simulink model "three_models_observer"  (R2021b)
settings: Solver=ode45  StartTime=0.0  StopTime=50  FixedStep=0.01  RelTol=1e-6  EnableMultiTasking=on
values from neighbouring files (symbols this model uses):
  a = -l^2+J/(mc+mp)    (= 0.00589092533208)    [parameters.m]    (also in simulation_models.m)
  A = [0 0 1 0;0 0 0 1;0 -l*mu*g/J -a*Fc/J -l*fp/J;0 -mu*g/J -l*Fc/J -fp/J]    [simulation_models.m]
  A1 = expm(A(2:4,2:4)*0.01)    [simulation_models.m]
  B = [0;0;a/J;l/J]    [simulation_models.m]
  B1 = (A1-eye(3))*inv(A(2:4,2:4))*B(2:4)    [simulation_models.m]
  C = [1 0 0 0;0 1 0 0;0 0 1 0;0 0 0 1]    [simulation_models.m]
  D = [0;0;0;0]    [simulation_models.m]
  DZcp = 6.8    [parameters.m]    (also in simulation_models.m)
  DZcv = 0.08    [parameters.m]    (also in simulation_models.m)
  DZu = 0.4    [parameters.m]    (also in simulation_models.m)
  Fc = 0.75    [parameters.m]    (also in simulation_models.m)
  FCD = 0.2501    [parameters.m]    (also in simulation_models.m)
  FCU = 0.8793    [parameters.m]    (also in simulation_models.m)
  fp = 0.0038    [parameters.m]    (also in simulation_models.m)
  FS = 2    [parameters.m]    (also in simulation_models.m)
  FSD = 2.7457    [parameters.m]    (also in simulation_models.m)
  FSdl = -1    [parameters.m]    (also in simulation_models.m)
  FSU = 2.7972    [parameters.m]    (also in simulation_models.m)
  FSul = 2    [parameters.m]    (also in simulation_models.m)
  g = 9.81    [parameters.m]    (also in simulation_models.m)
  J = 0.0075    [parameters.m]    (also in simulation_models.m)
  l = 0.0167903    [parameters.m]    (also in simulation_models.m)
  M = 22.304    [parameters.m]    (also in simulation_models.m)
  mu = l*(mc+mp)    (= 0.0204002145)    [parameters.m]    (also in simulation_models.m)
  Um = 0.5    [parameters.m]    (also in simulation_models.m)
  Xc = 2    [parameters.m]    (also in simulation_models.m)
  Yc = 2    [parameters.m]    (also in simulation_models.m)
undefined symbols (not defined in the file or in its folder): den, DiscIntNeverNeededParam, num
settings Model: Creator=ramon_perez  LastModifiedBy=szmis
settings SolverCC: AlgebraicLoopSolver=TrustRegion
settings DataIOCC: SaveFormat=Array  SignalLoggingSaveFormat=ModelDataLogs  ReturnWorkspaceOutputs=off
settings OptimizationCC: BlockReduction=off  BooleanDataType=off  ExpressionDepthLimit=2147483647  LifeSpan=inf
settings DebuggingCC: SaveWithParameterizedLinksMsg=none  UnderspecifiedInitializationDetection=Classic  MergeDetectMultiDrivingBlocksExec=none  SignalResolutionControl=TryResolveAllWithWarning  MultiTaskDSMMsg=warning  MultiTaskCondExecSysMsg=none  FcnCallInpInsideContextMsg=warning  StateNameClashWarn=warning  SFUnexpectedBacktrackingDiag=warning  SFNoUnconditionalDefaultTransitionDiag=warning  SFExecutionAtInitializationDiag=none  SFMachineParentedDataDiag=warning  ArithmeticOperatorsInVariantConditions=warning
settings HardwareCC: ProdBitPerPointer=32  ProdBitPerSizeT=32  ProdBitPerPtrDiffT=32  ProdLargestAtomicFloat=None  ProdIntDivRoundTo=Undefined  ProdEndianess=Unspecified  ProdWordSize=32  ProdHWDeviceType=32-bit Generic  TargetUnknown=on
settings ModelReferenceCC: PropagateSignalLabelsOutOfModel=off
settings SFSimCC: SimUseLocalCustomCode=off  CustomCodeUndefinedFunction=UseInterfaceOnly
settings RTWCC: RTWUseLocalCustomCode=off
settings CodeAppCC: StateflowObjectComments=on
settings GRTTargetCC: TargetLangStandard=C89/C90 (ANSI)  CombineOutputUpdateFcns=off  GRTInterface=on
settings ConfigComp: CovMetricSettings=dw  CovSaveCumulativeToWorkspaceVar=on  CovSaveSingleToWorkspaceVar=on  CovExternalEMLEnable=off

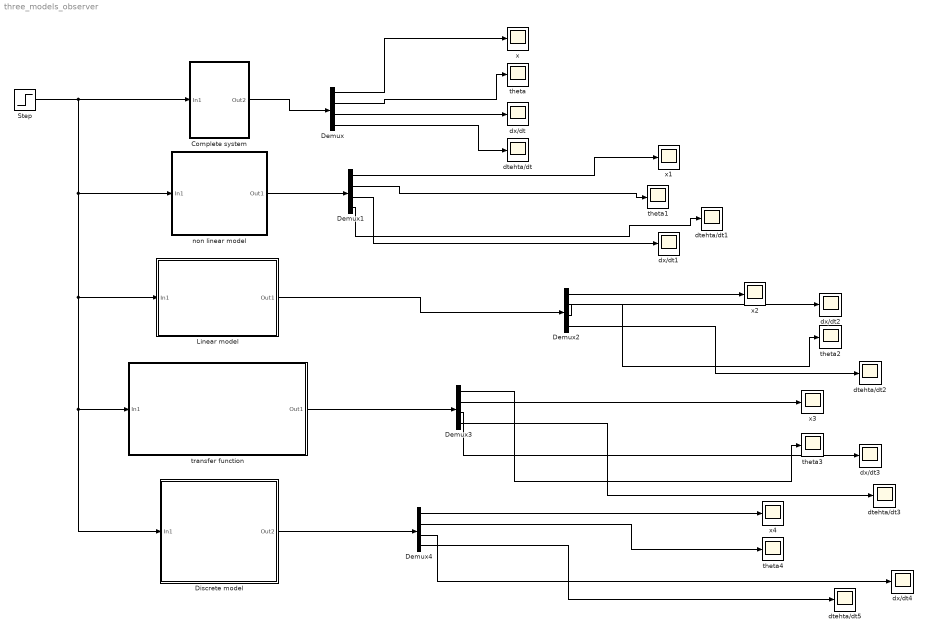
== system three_models_observer ==
  Complete system : Subsystem
  Demux{,1..4} (5 alike) : Demux
  Discrete model : Subsystem
  Linear model : Subsystem
  Step : Step  After=0.3  SampleTime=0
  dtehta/dt{,1..3,5} (5 alike) : Scope
  dx/dt{,1..4} (5 alike) : Scope
  non linear model : Subsystem
  theta{,1..4} (5 alike) : Scope
  transfer function : Subsystem
  x{,1..4} (5 alike) : Scope
  wires:
  Step/1 -> Complete system/1(In1), transfer function/1(In1), Discrete model/1(In1), Linear model/1(In1), non linear model/1(In1)
  Complete system/1(Out2) -> Demux/1
  Demux/1 -> x/1
  Demux/2 -> theta/1
  Demux/3 -> dx/dt/1
  Demux/4 -> dtehta/dt/1
  non linear model/1(Out1) -> Demux1/1
  Demux1/1 -> x1/1
  Demux1/2 -> theta1/1
  Demux1/3 -> dx/dt1/1
  Demux1/4 -> dtehta/dt1/1
  Linear model/1(Out1) -> Demux2/1
  Demux2/1 -> x2/1
  Demux2/2 -> theta2/1
  Demux2/3 -> dx/dt2/1
  Demux2/4 -> dtehta/dt2/1
  Demux3/1 -> x3/1
  Demux3/2 -> theta3/1
  Demux3/3 -> dx/dt3/1
  Demux3/4 -> dtehta/dt3/1
  transfer function/1(Out1) -> Demux3/1
  Demux4/1 -> x4/1
  Demux4/2 -> theta4/1
  Demux4/3 -> dx/dt4/1
  Demux4/4 -> dtehta/dt5/1
  Discrete model/1(Out2) -> Demux4/1

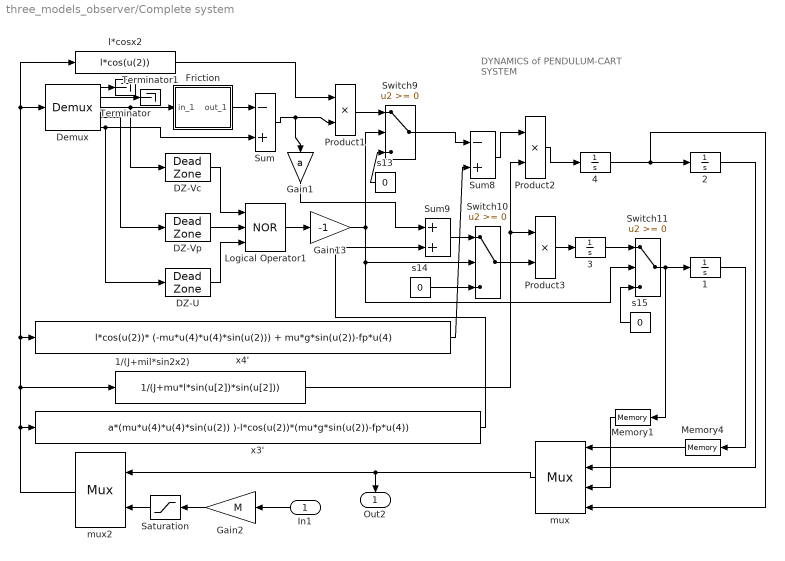
== system three_models_observer/Complete system ==
  note: DYNAMICS
      | of
      | PENDULUM-CART SYSTEM
  In1 : Inport
  1 : Integrator
  1/(J+mil*sin2x2) : Fcn  Expr=1/(J+mu*l*sin(u[2])*sin(u[2]))
  2 : Integrator  InitialCondition=pi
  3 : Integrator
  4 : Integrator
  DZ-U : DeadZone  LowerValue=-DZu  UpperValue=DZu  SaturateOnIntegerOverflow=on
  DZ-Vc : DeadZone  LowerValue=-DZcv  UpperValue=DZcv  SaturateOnIntegerOverflow=on
  DZ-Vp : DeadZone  LowerValue=-DZcp  UpperValue=DZcp  SaturateOnIntegerOverflow=on
  Demux : Demux  Outputs=5
      settings: DisplayOption=none
  Friction : Subsystem  mask(Friction model){FSD=FSD, FSU=FSU, FCD=FCD, FCU=FCU, FSdl=FSdl, FSul=FSul, FS=FS, Xc=Xc, Yc=Yc, small=DZcv}
      mask prompts: FSD "Static friction (FSD) [N]:"; FSU "Static friction (FSU) [N] :"; FCD "Columbic friction (FCD) [N]:"; FCU "Coulombic friction (FCU)  [N] :"; FSdl "Coulombic friction (FSdl) [N]:"; FSul "Coulombic friction (Fsul) [N]:"; FS "Coulombic friction (FS) [N]:"; Xc "Point for minimum (X1) [m/s] :"; Yc "Friction value for Xc point (Yc) [N] :"; small "Linear zone :"
      mask help: Friction implemented as nonlinear function. Copyright Adam PI£AT 1997.
      mask init:
      | Z=small;
      mask Help: Friction vs. cart velocity
      mask Display: plot(0,0,10,20,[1,9],[10,10],[5,5],[1,19],[0,1,2,3,4,5],[7,7.5,8,8.5,8.3,3],[5,6,7,8,9,10],[17,11.7,11.5,12,12.5,13])
  Gain1 : Gain  Gain=a  SaturateOnIntegerOverflow=on  OutDataTypeStr=Inherit: Same as input  ParamDataTypeStr=Inherit: Same as input
  Gain13 : Gain  Gain=-1  SaturateOnIntegerOverflow=on  OutDataTypeStr=Inherit: Same as input  ParamDataTypeStr=Inherit: Same as input
  Gain2 : Gain  Gain=M  OutDataTypeStr=Inherit: Same as input  ParamDataTypeStr=Inherit: Same as input
  Logical Operator1 : Logic  Operator=NOR  Inputs=3
  Memory1 : Memory
  Memory4 : Memory
  Product1 : Product  InputSameDT=on  RndMeth=Zero  SaturateOnIntegerOverflow=on  OutDataTypeStr=Inherit: Same as first input
  Product2 : Product  InputSameDT=on  RndMeth=Zero  SaturateOnIntegerOverflow=on  OutDataTypeStr=Inherit: Same as first input
  Product3 : Product  InputSameDT=on  RndMeth=Zero  SaturateOnIntegerOverflow=on  OutDataTypeStr=Inherit: Same as first input
  Saturation : Saturate  UpperLimit=Um*M  LowerLimit=-Um*M
  Sum : Sum  Inputs=-+  InputSameDT=on  SaturateOnIntegerOverflow=on  OutDataTypeStr=Inherit: Same as first input
  Sum8 : Sum  Inputs=-+  InputSameDT=on  SaturateOnIntegerOverflow=on  OutDataTypeStr=Inherit: Same as first input
  Sum9 : Sum  InputSameDT=on  SaturateOnIntegerOverflow=on  OutDataTypeStr=Inherit: Same as first input
  Switch10 : Switch  SaturateOnIntegerOverflow=on  InputSameDT=on
  Switch11 : Switch  SaturateOnIntegerOverflow=on  InputSameDT=on
  Switch9 : Switch  SaturateOnIntegerOverflow=on  InputSameDT=on
  Terminator : Terminator
  Terminator1 : Terminator
  l*cosx2 : Fcn  Expr=l*cos(u(2))
  mux : Mux
  mux2 : Mux  Inputs=[4 1]
  s13 : Constant  Value=0
  s14 : Constant  Value=0
  s15 : Constant  Value=0
  x3' : Fcn  Expr=a*(mu*u(4)*u(4)*sin(u(2)) )-l*cos(u(2))*(mu*g*sin(u(2))-fp*u(4))
  x4' : Fcn  Expr=l*cos(u(2))* (-mu*u(4)*u(4)*sin(u(2))) + mu*g*sin(u(2))-fp*u(4)
  Out2 : Outport
  wires:
  Demux/2 -> Terminator1/1
  Demux/1 -> Terminator/1
  l*cosx2/1 -> Product1/1
  DZ-U/1 -> Logical Operator1/3
  DZ-Vp/1 -> Logical Operator1/2
  DZ-Vc/1 -> Logical Operator1/1
  Logical Operator1/1 -> Gain13/1
  s13/1 -> Switch9/3
  Switch9/1 -> Sum8/1
  s14/1 -> Switch10/3
  Product1/1 -> Switch9/1
  x4'/1 -> Sum8/2
  Sum8/1 -> Product2/1
  Product2/1 -> 4/1
  Product3/1 -> 3/1
  Demux/3 -> Friction/1(in_1), DZ-Vc/1
  Demux/4 -> DZ-Vp/1
  Sum9/1 -> Switch10/1
  s15/1 -> Switch11/3
  Memory1/1 -> mux/3
  Switch11/1 -> 1/1, Memory1/1
  Saturation/1 -> mux2/2
  Gain2/1 -> Saturation/1
  Friction/1(out_1) -> Sum/1
  Gain13/1 -> Switch9/2, Switch11/2, Switch10/2
  Demux/5 -> Sum/2, DZ-U/1
  Switch10/1 -> Product3/2
  Sum/1 -> Product1/2, Gain1/1
  Gain1/1 -> Sum9/1
  mux2/1 -> x3'/1, l*cosx2/1, Demux/1, x4'/1, 1/(J+mil*sin2x2)/1
  x3'/1 -> Sum9/2
  1/(J+mil*sin2x2)/1 -> Product2/2, Product3/1
  1/1 -> Memory4/1
  Memory4/1 -> mux/1
  4/1 -> 2/1, mux/4
  3/1 -> Switch11/1
  In1/1 -> Gain2/1
  mux/1 -> mux2/1, Out2/1
  2/1 -> mux/2

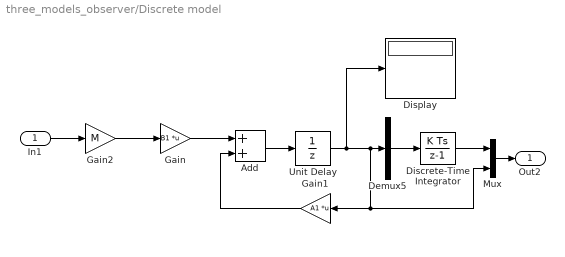
== system three_models_observer/Discrete model ==
  In1 : Inport
  Add : Sum
  Demux5 : Demux  Outputs=3
  Discrete-Time Integrator : DiscreteIntegrator  SampleTime=0.1  ICPrevOutput=DiscIntNeverNeededParam  ICPrevScaledInput=DiscIntNeverNeededParam
  Display : Display
  Gain : Gain  Gain=B1  Multiplication=Matrix(K*u)  SampleTime=0.1
  Gain1 : Gain  Gain=A1  Multiplication=Matrix(K*u)  SampleTime=0.1
  Gain2 : Gain  Gain=M  SampleTime=0.1
  Mux : Mux  Inputs=2
  Unit Delay : UnitDelay  SampleTime=0.1  HasFrameUpgradeWarning=on
  Out2 : Outport
  wires:
  Add/1 -> Unit Delay/1
  Gain/1 -> Add/1
  Gain1/1 -> Add/2
  Unit Delay/1 -> Display/1, Demux5/1, Gain1/1, Mux/2
  Gain2/1 -> Gain/1
  Discrete-Time Integrator/1 -> Mux/1
  Demux5/2 -> Discrete-Time Integrator/1
  In1/1 -> Gain2/1
  Mux/1 -> Out2/1

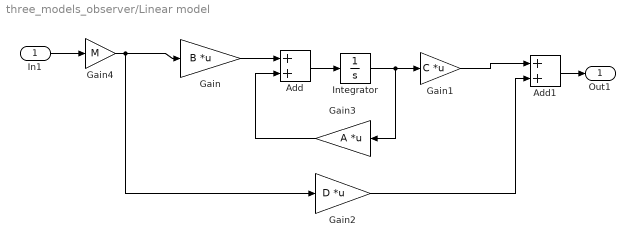
== system three_models_observer/Linear model ==
  In1 : Inport
  Add : Sum
  Add1 : Sum
  Gain : Gain  Gain=B  Multiplication=Matrix(K*u)
  Gain1 : Gain  Gain=C  Multiplication=Matrix(K*u)
  Gain2 : Gain  Gain=D  Multiplication=Matrix(K*u)
  Gain3 : Gain  Gain=A  Multiplication=Matrix(K*u)
  Gain4 : Gain  Gain=M
  Integrator : Integrator
  Out1 : Outport
  wires:
  Add/1 -> Integrator/1
  Gain/1 -> Add/1
  Gain3/1 -> Add/2
  Integrator/1 -> Gain1/1, Gain3/1
  Gain1/1 -> Add1/1
  Gain2/1 -> Add1/2
  Gain4/1 -> Gain/1, Gain2/1
  In1/1 -> Gain4/1
  Add1/1 -> Out1/1

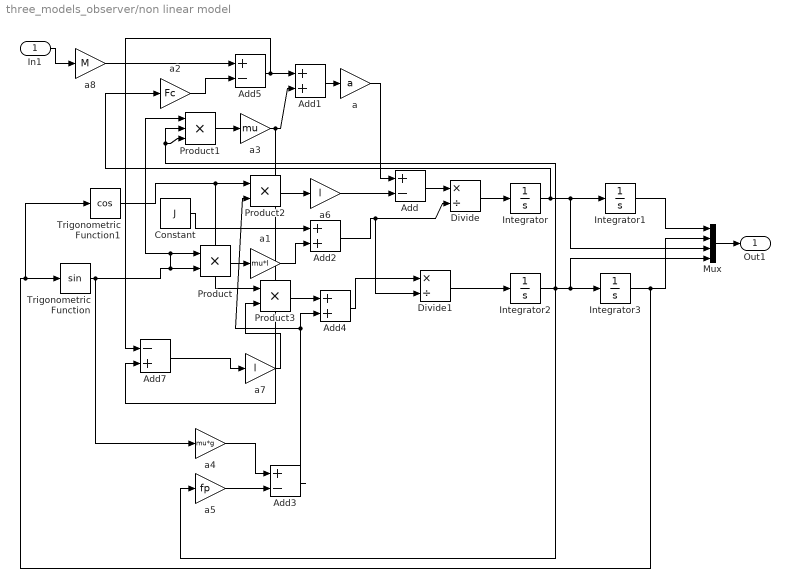
== system three_models_observer/non linear model ==
  In1 : Inport
  Add : Sum  Inputs=+-
  Add1 : Sum
  Add2 : Sum
  Add3 : Sum  Inputs=+-
  Add4 : Sum
  Add5 : Sum  Inputs=+-
  Add7 : Sum  Inputs=-+
  Constant : Constant  Value=J
  Divide : Product  Inputs=*/
  Divide1 : Product  Inputs=*/
  Integrator : Integrator
  Integrator1 : Integrator
  Integrator2 : Integrator
  Integrator3 : Integrator  InitialCondition=pi
  Mux : Mux
  Product : Product  RndMeth=Zero
  Product1 : Product  Inputs=3  RndMeth=Zero
  Product2 : Product  RndMeth=Zero
  Product3 : Product  RndMeth=Zero
  Trigonometric Function : Trigonometry
  Trigonometric Function1 : Trigonometry  Operator=cos
  a : Gain  Gain=a
  a1 : Gain  Gain=mu*l
  a2 : Gain  Gain=Fc
  a3 : Gain  Gain=mu
  a4 : Gain  Gain=mu*g
  a5 : Gain  Gain=fp
  a6 : Gain  Gain=l
  a7 : Gain  Gain=l
  a8 : Gain  Gain=M
  Out1 : Outport
  wires:
  Integrator/1 -> Integrator1/1, Mux/3, a2/1
  Integrator2/1 -> Integrator3/1, Mux/4, Product1/2, Product1/3, a5/1
  Integrator1/1 -> Mux/1
  Integrator3/1 -> Mux/2, Trigonometric Function/1, Trigonometric Function1/1
  Divide1/1 -> Integrator2/1
  Divide/1 -> Integrator/1
  a/1 -> Add/1
  Add/1 -> Divide/1
  Add1/1 -> a/1
  Add2/1 -> Divide/2, Divide1/2
  Constant/1 -> Add2/1
  Trigonometric Function/1 -> Product/2, Product/1, Product1/1, a4/1
  a1/1 -> Add2/2
  Product1/1 -> a3/1
  a3/1 -> Add1/2, Add7/2
  Add4/1 -> Divide1/1
  Add3/1 -> Add4/2, Product2/2
  a4/1 -> Add3/1
  a5/1 -> Add3/2
  Product/1 -> a1/1
  Add5/1 -> Add1/1, Add7/1
  a2/1 -> Add5/2
  a6/1 -> Add/2
  Product2/1 -> a6/1
  Trigonometric Function1/1 -> Product2/1, Product3/1
  Add7/1 -> a7/1
  Product3/1 -> Add4/1
  a7/1 -> Product3/2
  In1/1 -> a8/1
  Mux/1 -> Out1/1
  a8/1 -> Add5/1

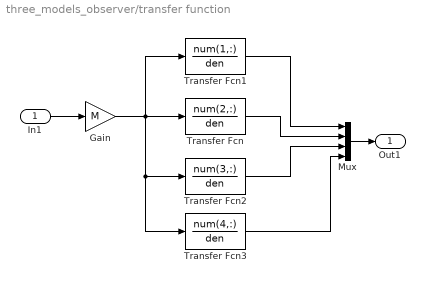
== system three_models_observer/transfer function ==
  In1 : Inport
  Gain : Gain  Gain=M
  Mux : Mux
  Transfer Fcn : TransferFcn  Numerator=num(2,:)  Denominator=den
  Transfer Fcn1 : TransferFcn  Numerator=num(1,:)  Denominator=den
  Transfer Fcn2 : TransferFcn  Numerator=num(3,:)  Denominator=den
  Transfer Fcn3 : TransferFcn  Numerator=num(4,:)  Denominator=den
  Out1 : Outport
  wires:
  Gain/1 -> Transfer Fcn3/1, Transfer Fcn2/1, Transfer Fcn1/1, Transfer Fcn/1
  Transfer Fcn1/1 -> Mux/1
  Transfer Fcn/1 -> Mux/2
  Transfer Fcn2/1 -> Mux/3
  Transfer Fcn3/1 -> Mux/4
  In1/1 -> Gain/1
  Mux/1 -> Out1/1

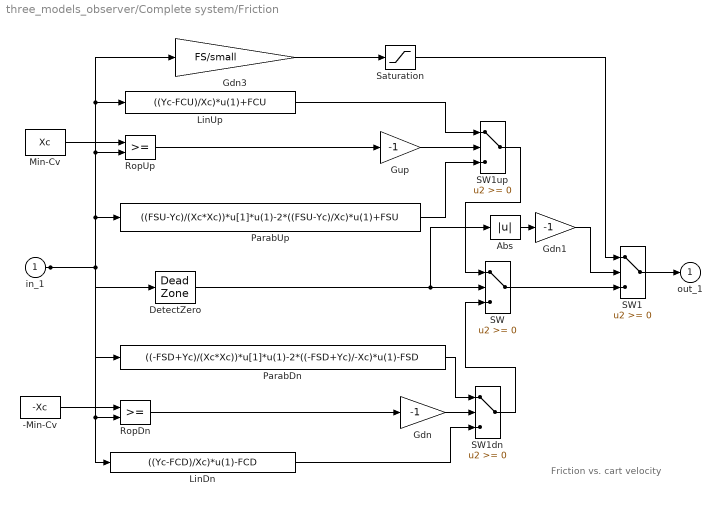
== system three_models_observer/Complete system/Friction ==
  note: Friction vs. cart velocity
  in_1 : Inport
  -Min-Cv : Constant  Value=-Xc
  Abs : Abs  SaturateOnIntegerOverflow=on
  DetectZero : DeadZone  LowerValue=-Z  UpperValue=Z  SaturateOnIntegerOverflow=on
  Gdn : Gain  Gain=-1  SaturateOnIntegerOverflow=on  OutDataTypeStr=Inherit: Same as input  ParamDataTypeStr=Inherit: Same as input
  Gdn1 : Gain  Gain=-1  SaturateOnIntegerOverflow=on  OutDataTypeStr=Inherit: Same as input  ParamDataTypeStr=Inherit: Same as input
  Gdn3 : Gain  Gain=FS/small  SaturateOnIntegerOverflow=on  OutDataTypeStr=Inherit: Same as input  ParamDataTypeStr=Inherit: Same as input
  Gup : Gain  Gain=-1  SaturateOnIntegerOverflow=on  OutDataTypeStr=Inherit: Same as input  ParamDataTypeStr=Inherit: Same as input
  LinDn : Fcn  Expr=((Yc-FCD)/Xc)*u(1)-FCD
  LinUp : Fcn  Expr=((Yc-FCU)/Xc)*u(1)+FCU
  Min-Cv : Constant  Value=Xc
  ParabDn : Fcn  Expr=((-FSD+Yc)/(Xc*Xc))*u[1]*u(1)-2*((-FSD+Yc)/-Xc)*u(1)-FSD
  ParabUp : Fcn  Expr=((FSU-Yc)/(Xc*Xc))*u[1]*u(1)-2*((FSU-Yc)/Xc)*u(1)+FSU
  RopDn : RelationalOperator  RndMeth=Nearest  InputSameDT=on
  RopUp : RelationalOperator  RndMeth=Nearest  InputSameDT=on
  SW : Switch  SaturateOnIntegerOverflow=on  InputSameDT=on
  SW1 : Switch  SaturateOnIntegerOverflow=on  InputSameDT=on
  SW1dn : Switch  SaturateOnIntegerOverflow=on  InputSameDT=on
  SW1up : Switch  SaturateOnIntegerOverflow=on  InputSameDT=on
  Saturation : Saturate  UpperLimit=FSul  LowerLimit=FSdl
  out_1 : Outport  InitialOutput=0
  wires:
  Saturation/1 -> SW1/1
  Gdn3/1 -> Saturation/1
  in_1/1 -> RopUp/2, LinUp/1, Gdn3/1, ParabUp/1, ParabDn/1, DetectZero/1, LinDn/1, RopDn/2
  SW1/1 -> out_1/1
  DetectZero/1 -> SW/2, Abs/1
  Gdn1/1 -> SW1/2
  Abs/1 -> Gdn1/1
  SW/1 -> SW1/3
  Min-Cv/1 -> RopUp/1
  RopUp/1 -> Gup/1
  Gup/1 -> SW1up/2
  ParabUp/1 -> SW1up/3
  LinUp/1 -> SW1up/1
  SW1up/1 -> SW/1
  -Min-Cv/1 -> RopDn/1
  RopDn/1 -> Gdn/1
  Gdn/1 -> SW1dn/2
  LinDn/1 -> SW1dn/3
  ParabDn/1 -> SW1dn/1
  SW1dn/1 -> SW/3
